simulink model "semi_active_suspension_mr_damper_full_vehicle"  (R2022b)
settings: Solver=ode1be  StartTime=0.0  StopTime=120  FixedStep=0.001  RelTol=1e-3
model workspace (MAT data in the model file):
  D_common1 = 500
  I_common = 50
  P_common = 4000
  a1 = 1.6
  a2 = 1.6
  a3 = 1.4
  a4 = 1.4
  filter_coefficient = 2000
  mr_damper_base_damping = 500
  s1 = 0.78
  s2 = 0.78
  s3 = 0.79
  s4 = 0.79
libraries: slpidlib x4
settings Model: Creator=giris  LastModifiedBy=giris

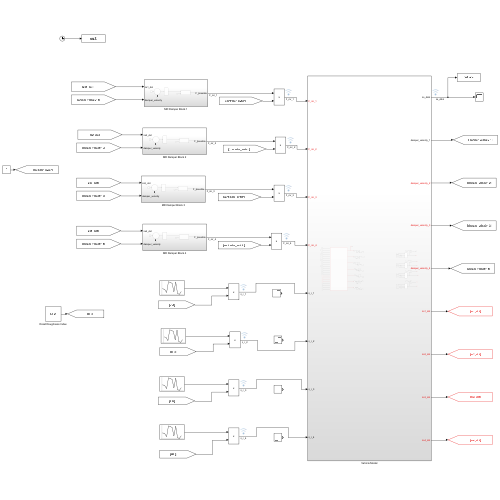
[thumbnail: Simulink's stored preview of the top-level diagram]
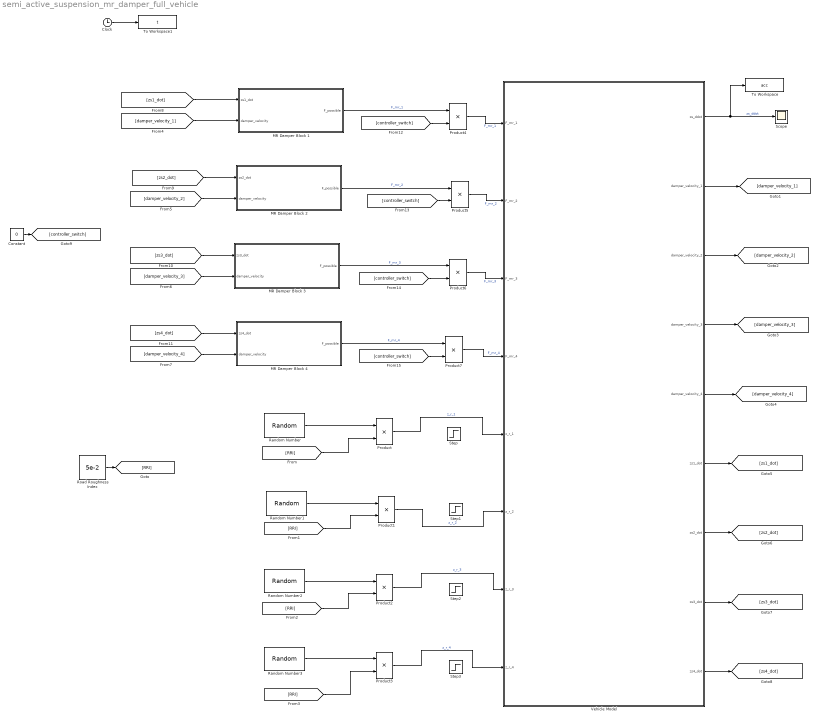
== system semi_active_suspension_mr_damper_full_vehicle ==
  Clock : Clock
  Constant : Constant  Value=0
  MR Damper Block 1 : Subsystem
  MR Damper Block 2 : Subsystem
  MR Damper Block 3 : Subsystem
  MR Damper Block 4 : Subsystem
  Product{,1..7} (8 alike) : Product
  Random Number : RandomNumber  SampleTime=0.01
  Random Number1 : RandomNumber  Seed=1  SampleTime=0.01
  Random Number2 : RandomNumber  Seed=2  SampleTime=0.01
  Random Number3 : RandomNumber  Seed=3  SampleTime=0.01
  Road Roughness Index : Constant  Value=5e-2
  Scope : Scope
  Step : Step  After=0.01  SampleTime=0
  Step1 : Step  After=0.01  SampleTime=0
  Step2 : Step  Time=1.135  After=0.01  SampleTime=0
  Step3 : Step  Time=1.135  After=0.01  SampleTime=0
  To Workspace : ToWorkspace  VariableName=acc  SaveFormat=Timeseries  SampleTime=-1
  To Workspace1 : ToWorkspace  VariableName=t  SaveFormat=Timeseries  SampleTime=-1
  Vehicle Model : Subsystem
  wires:
  MR Damper Block 3/1(F_possible) -> Product6/1  "F_mr_3"
  Random Number2/1 -> Product2/1
  Random Number/1 -> Product/1
  MR Damper Block 4/1(F_possible) -> Product7/1  "F_mr_4"
  Random Number1/1 -> Product1/1
  Random Number3/1 -> Product3/1
  MR Damper Block 1/1(F_possible) -> Product4/1  "F_mr_1"
  MR Damper Block 2/1(F_possible) -> Product5/1  "F_mr_2"
  Vehicle Model/1(zs_ddot) -> To Workspace/1, Scope/1  "zs_ddot"
  Road Roughness Index/1 -> [RRI]
  [RRI] -> Product/2
  [RRI] -> Product2/2
  [RRI] -> Product3/2
  [RRI] -> Product1/2
  Vehicle Model/5(damper_velocity_4) -> [damper_velocity_4]
  Vehicle Model/4(damper_velocity_3) -> [damper_velocity_3]
  Vehicle Model/3(damper_velocity_2) -> [damper_velocity_2]
  [damper_velocity_1] -> MR Damper Block 1/2(damper_velocity)
  [damper_velocity_2] -> MR Damper Block 2/2(damper_velocity)
  [damper_velocity_3] -> MR Damper Block 3/2(damper_velocity)
  [damper_velocity_4] -> MR Damper Block 4/2(damper_velocity)
  Vehicle Model/6(zs1_dot) -> [zs1_dot]
  Vehicle Model/7(zs2_dot) -> [zs2_dot]
  Vehicle Model/8(zs3_dot) -> [zs3_dot]
  Vehicle Model/9(zs4_dot) -> [zs4_dot]
  [zs1_dot] -> MR Damper Block 1/1(zs1_dot)
  [zs2_dot] -> MR Damper Block 2/1(zs2_dot)
  [zs3_dot] -> MR Damper Block 3/1(zs3_dot)
  [zs4_dot] -> MR Damper Block 4/1(zs4_dot)
  Product4/1 -> Vehicle Model/1(F_mr_1)  "F_mr_1"
  Product5/1 -> Vehicle Model/2(F_mr_2)  "F_mr_2"
  Product6/1 -> Vehicle Model/3(F_mr_3)  "F_mr_3"
  Product7/1 -> Vehicle Model/4(F_mr_4)  "F_mr_4"
  Constant/1 -> [controller_switch]
  [controller_switch] -> Product4/2
  [controller_switch] -> Product5/2
  [controller_switch] -> Product6/2
  [controller_switch] -> Product7/2
  Vehicle Model/2(damper_velocity_1) -> [damper_velocity_1]
  Clock/1 -> To Workspace1/1
  Product/1 -> Vehicle Model/5(z_r_1)  "z_r_1"
  Product1/1 -> Vehicle Model/6(z_r_2)  "z_r_2"
  Product2/1 -> Vehicle Model/7(z_r_3)  "z_r_3"
  Product3/1 -> Vehicle Model/8(z_r_4)  "z_r_4"

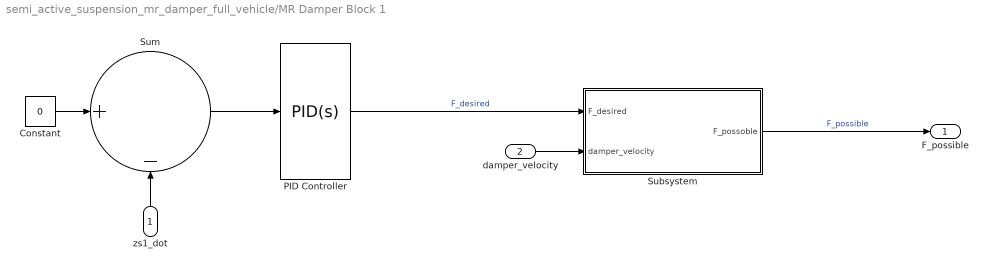
== system semi_active_suspension_mr_damper_full_vehicle/MR Damper Block 1 ==
  zs1_dot : Inport
  damper_velocity : Inport  Port=2
  Constant : Constant  Value=0
  PID Controller : slpidlib/PID Controller  Controller=PID  Form=Parallel  TimeDomain=Continuous-time  UseExternalTs=off  SampleTime=-1  IntegratorMethod=Forward Euler  FilterMethod=Forward Euler  ControllerParametersSource=internal  P=P_common  I=I_common  UseKiTs=off  D=D_common1  N=filter_coefficient  UseFilter=on  TunerSelectOption=Transfer Function Based (PID Tuner App)  InitialConditionSource=internal  InitialConditionForIntegrator=0  InitialConditionForFilter=0  DifferentiatorICPrevScaledInput=0  ExternalReset=none  TrackingMode=off  Kt=1  LimitOutput=off  SatLimitsSource=internal  UpperSaturationLimit=inf  LowerSaturationLimit=-inf  LinearizeAsGain=on  AntiWindupMode=none  Kb=1  LimitIntegrator=off  UpperIntegratorSaturationLimit=inf  LowerIntegratorSaturationLimit=-inf  POutMin=[]  POutMax=[]  IOutMin=[]  IOutMax=[]  DOutMin=[]  DOutMax=[]  NOutMin=[]  NOutMax=[]  SumOutMin=[]  SumOutMax=[]  SaturationOutMin=[]  SaturationOutMax=[]  PParamMin=[]  PParamMax=[]  IParamMin=[]  IParamMax=[]  DParamMin=[]  DParamMax=[]  NParamMin=[]  NParamMax=[]  KbParamMin=[]  KbParamMax=[]  KtParamMin=[]  KtParamMax=[]  KbOutMin=[]  KbOutMax=[]  KtOutMin=[]  KtOutMax=[]  IntegratorOutMin=[]  IntegratorOutMax=[]  FilterOutMin=[]  FilterOutMax=[]  SumI1OutMin=[]  SumI1OutMax=[]  SumI2OutMin=[]  SumI2OutMax=[]  SumI3OutMin=[]  SumI3OutMax=[]  SumI4OutMin=[]  SumI4OutMax=[]  SumDOutMin=[]  SumDOutMax=[]  DifferentiatorOutMin=[]  DifferentiatorOutMax=[]  FilterDiffOutCoefMin=[]  FilterDiffOutCoefMax=[]  ReciprocalOutMin=[]  ReciprocalOutMax=[]  SumDenOutMin=[]  SumDenOutMax=[]  SumNumOutMin=[]  SumNumOutMax=[]  DivideOutMin=[]  DivideOutMax=[]  UdiffTsProdOutMin=[]  UdiffTsProdOutMax=[]  NTsProdOutMin=[]  NTsProdOutMax=[]  UintegralTsProdOutMin=[]  UintegralTsProdOutMax=[]  UngainTsProdOutMin=[]  UngainTsProdOutMax=[]  ClampingZeroOutDataTypeStr=Inherit: Inherit via back propagation  ClampingZeroOutMin=[]  ClampingZeroOutMax=[]  FilterDenConstantOutDataTypeStr=Inherit: Inherit via back propagation  FilterDenConstantOutMin=[]  FilterDenConstantOutMax=[]  PCopyOutDataTypeStr=Inherit: Inherit via back propagation  PCopyOutMin=[]  PCopyOutMax=[]  NCopyOutDataTypeStr=Inherit: Inherit via back propagation  NCopyOutMin=[]  NCopyOutMax=[]  IntegratorContinuousStateAttributes=''  IntegratorStateMustResolveToSignalObject=off  IntegratorRTWStateStorageClass=Auto  FilterContinuousStateAttributes=''  FilterStateMustResolveToSignalObject=off  FilterRTWStateStorageClass=Auto  ParallelPVariant=InternalParameters  IdealPVariant=Disabled  IVariant=InternalParameters  DVariant=InternalParameters  IntegratorVariant=Continuous  SatVariant=Disabled  AWVariant=Passthrough  PCopyVariant=Disabled  TRVariant=Disabled  FdbkBlocksVariant=Forward  IdealPFdbkVariant=Disabled  SatFdbkVariant=Disabled  DerivativeFilterVariant=ContFilter  NVariant=InternalParameters  NCopyVariant=Disabled  FilterICVariant=InternalICsFilter  IntegratorICVariant=InternalICs  ExternalResetVariant=Disabled  TRSumVariant=Passthrough  SumFdbkVariant=Disabled  SumVariant=Sum_PID  TsampFilterVariant=InternalTs  TsampNgainVariant=Passthrough  TsampIntegralVariant=Passthrough  ExternalSaturationOutDataTypeStr=Inherit: Same as second input
  Subsystem : Subsystem
  Sum : Sum  Inputs=|+-
  F_possible : Outport
  wires:
  PID Controller/1 -> Subsystem/1(F_desired)  "F_desired"
  Subsystem/1(F_possoble) -> F_possible/1  "F_possible"
  Sum/1 -> PID Controller/1
  Constant/1 -> Sum/1
  zs1_dot/1 -> Sum/2
  damper_velocity/1 -> Subsystem/2(damper_velocity)

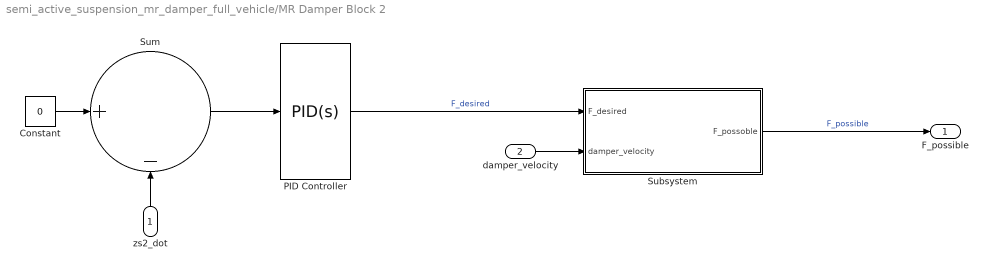
== system semi_active_suspension_mr_damper_full_vehicle/MR Damper Block 2 ==
  zs2_dot : Inport
  damper_velocity : Inport  Port=2
  Constant : Constant  Value=0
  PID Controller : slpidlib/PID Controller  Controller=PID  Form=Parallel  TimeDomain=Continuous-time  UseExternalTs=off  SampleTime=-1  IntegratorMethod=Forward Euler  FilterMethod=Forward Euler  ControllerParametersSource=internal  P=P_common  I=I_common  UseKiTs=off  D=D_common1  N=filter_coefficient  UseFilter=on  TunerSelectOption=Transfer Function Based (PID Tuner App)  InitialConditionSource=internal  InitialConditionForIntegrator=0  InitialConditionForFilter=0  DifferentiatorICPrevScaledInput=0  ExternalReset=none  TrackingMode=off  Kt=1  LimitOutput=off  SatLimitsSource=internal  UpperSaturationLimit=inf  LowerSaturationLimit=-inf  LinearizeAsGain=on  AntiWindupMode=none  Kb=1  LimitIntegrator=off  UpperIntegratorSaturationLimit=inf  LowerIntegratorSaturationLimit=-inf  POutMin=[]  POutMax=[]  IOutMin=[]  IOutMax=[]  DOutMin=[]  DOutMax=[]  NOutMin=[]  NOutMax=[]  SumOutMin=[]  SumOutMax=[]  SaturationOutMin=[]  SaturationOutMax=[]  PParamMin=[]  PParamMax=[]  IParamMin=[]  IParamMax=[]  DParamMin=[]  DParamMax=[]  NParamMin=[]  NParamMax=[]  KbParamMin=[]  KbParamMax=[]  KtParamMin=[]  KtParamMax=[]  KbOutMin=[]  KbOutMax=[]  KtOutMin=[]  KtOutMax=[]  IntegratorOutMin=[]  IntegratorOutMax=[]  FilterOutMin=[]  FilterOutMax=[]  SumI1OutMin=[]  SumI1OutMax=[]  SumI2OutMin=[]  SumI2OutMax=[]  SumI3OutMin=[]  SumI3OutMax=[]  SumI4OutMin=[]  SumI4OutMax=[]  SumDOutMin=[]  SumDOutMax=[]  DifferentiatorOutMin=[]  DifferentiatorOutMax=[]  FilterDiffOutCoefMin=[]  FilterDiffOutCoefMax=[]  ReciprocalOutMin=[]  ReciprocalOutMax=[]  SumDenOutMin=[]  SumDenOutMax=[]  SumNumOutMin=[]  SumNumOutMax=[]  DivideOutMin=[]  DivideOutMax=[]  UdiffTsProdOutMin=[]  UdiffTsProdOutMax=[]  NTsProdOutMin=[]  NTsProdOutMax=[]  UintegralTsProdOutMin=[]  UintegralTsProdOutMax=[]  UngainTsProdOutMin=[]  UngainTsProdOutMax=[]  ClampingZeroOutDataTypeStr=Inherit: Inherit via back propagation  ClampingZeroOutMin=[]  ClampingZeroOutMax=[]  FilterDenConstantOutDataTypeStr=Inherit: Inherit via back propagation  FilterDenConstantOutMin=[]  FilterDenConstantOutMax=[]  PCopyOutDataTypeStr=Inherit: Inherit via back propagation  PCopyOutMin=[]  PCopyOutMax=[]  NCopyOutDataTypeStr=Inherit: Inherit via back propagation  NCopyOutMin=[]  NCopyOutMax=[]  IntegratorContinuousStateAttributes=''  IntegratorStateMustResolveToSignalObject=off  IntegratorRTWStateStorageClass=Auto  FilterContinuousStateAttributes=''  FilterStateMustResolveToSignalObject=off  FilterRTWStateStorageClass=Auto  ParallelPVariant=InternalParameters  IdealPVariant=Disabled  IVariant=InternalParameters  DVariant=InternalParameters  IntegratorVariant=Continuous  SatVariant=Disabled  AWVariant=Passthrough  PCopyVariant=Disabled  TRVariant=Disabled  FdbkBlocksVariant=Forward  IdealPFdbkVariant=Disabled  SatFdbkVariant=Disabled  DerivativeFilterVariant=ContFilter  NVariant=InternalParameters  NCopyVariant=Disabled  FilterICVariant=InternalICsFilter  IntegratorICVariant=InternalICs  ExternalResetVariant=Disabled  TRSumVariant=Passthrough  SumFdbkVariant=Disabled  SumVariant=Sum_PID  TsampFilterVariant=InternalTs  TsampNgainVariant=Passthrough  TsampIntegralVariant=Passthrough  ExternalSaturationOutDataTypeStr=Inherit: Same as second input
  Subsystem : Subsystem
  Sum : Sum  Inputs=|+-
  F_possible : Outport
  wires:
  damper_velocity/1 -> Subsystem/2(damper_velocity)
  zs2_dot/1 -> Sum/2
  Constant/1 -> Sum/1
  Sum/1 -> PID Controller/1
  Subsystem/1(F_possoble) -> F_possible/1  "F_possible"
  PID Controller/1 -> Subsystem/1(F_desired)  "F_desired"

== system semi_active_suspension_mr_damper_full_vehicle/MR Damper Block 3 ==
  zs3_dot : Inport
  damper_velocity : Inport  Port=2
  Constant : Constant  Value=0
  PID Controller : slpidlib/PID Controller  Controller=PID  Form=Parallel  TimeDomain=Continuous-time  UseExternalTs=off  SampleTime=-1  IntegratorMethod=Forward Euler  FilterMethod=Forward Euler  ControllerParametersSource=internal  P=P_common  I=I_common  UseKiTs=off  D=D_common1  N=filter_coefficient  UseFilter=on  TunerSelectOption=Transfer Function Based (PID Tuner App)  InitialConditionSource=internal  InitialConditionForIntegrator=0  InitialConditionForFilter=0  DifferentiatorICPrevScaledInput=0  ExternalReset=none  TrackingMode=off  Kt=1  LimitOutput=off  SatLimitsSource=internal  UpperSaturationLimit=inf  LowerSaturationLimit=-inf  LinearizeAsGain=on  AntiWindupMode=none  Kb=1  LimitIntegrator=off  UpperIntegratorSaturationLimit=inf  LowerIntegratorSaturationLimit=-inf  POutMin=[]  POutMax=[]  IOutMin=[]  IOutMax=[]  DOutMin=[]  DOutMax=[]  NOutMin=[]  NOutMax=[]  SumOutMin=[]  SumOutMax=[]  SaturationOutMin=[]  SaturationOutMax=[]  PParamMin=[]  PParamMax=[]  IParamMin=[]  IParamMax=[]  DParamMin=[]  DParamMax=[]  NParamMin=[]  NParamMax=[]  KbParamMin=[]  KbParamMax=[]  KtParamMin=[]  KtParamMax=[]  KbOutMin=[]  KbOutMax=[]  KtOutMin=[]  KtOutMax=[]  IntegratorOutMin=[]  IntegratorOutMax=[]  FilterOutMin=[]  FilterOutMax=[]  SumI1OutMin=[]  SumI1OutMax=[]  SumI2OutMin=[]  SumI2OutMax=[]  SumI3OutMin=[]  SumI3OutMax=[]  SumI4OutMin=[]  SumI4OutMax=[]  SumDOutMin=[]  SumDOutMax=[]  DifferentiatorOutMin=[]  DifferentiatorOutMax=[]  FilterDiffOutCoefMin=[]  FilterDiffOutCoefMax=[]  ReciprocalOutMin=[]  ReciprocalOutMax=[]  SumDenOutMin=[]  SumDenOutMax=[]  SumNumOutMin=[]  SumNumOutMax=[]  DivideOutMin=[]  DivideOutMax=[]  UdiffTsProdOutMin=[]  UdiffTsProdOutMax=[]  NTsProdOutMin=[]  NTsProdOutMax=[]  UintegralTsProdOutMin=[]  UintegralTsProdOutMax=[]  UngainTsProdOutMin=[]  UngainTsProdOutMax=[]  ClampingZeroOutDataTypeStr=Inherit: Inherit via back propagation  ClampingZeroOutMin=[]  ClampingZeroOutMax=[]  FilterDenConstantOutDataTypeStr=Inherit: Inherit via back propagation  FilterDenConstantOutMin=[]  FilterDenConstantOutMax=[]  PCopyOutDataTypeStr=Inherit: Inherit via back propagation  PCopyOutMin=[]  PCopyOutMax=[]  NCopyOutDataTypeStr=Inherit: Inherit via back propagation  NCopyOutMin=[]  NCopyOutMax=[]  IntegratorContinuousStateAttributes=''  IntegratorStateMustResolveToSignalObject=off  IntegratorRTWStateStorageClass=Auto  FilterContinuousStateAttributes=''  FilterStateMustResolveToSignalObject=off  FilterRTWStateStorageClass=Auto  ParallelPVariant=InternalParameters  IdealPVariant=Disabled  IVariant=InternalParameters  DVariant=InternalParameters  IntegratorVariant=Continuous  SatVariant=Disabled  AWVariant=Passthrough  PCopyVariant=Disabled  TRVariant=Disabled  FdbkBlocksVariant=Forward  IdealPFdbkVariant=Disabled  SatFdbkVariant=Disabled  DerivativeFilterVariant=ContFilter  NVariant=InternalParameters  NCopyVariant=Disabled  FilterICVariant=InternalICsFilter  IntegratorICVariant=InternalICs  ExternalResetVariant=Disabled  TRSumVariant=Passthrough  SumFdbkVariant=Disabled  SumVariant=Sum_PID  TsampFilterVariant=InternalTs  TsampNgainVariant=Passthrough  TsampIntegralVariant=Passthrough  ExternalSaturationOutDataTypeStr=Inherit: Same as second input
  Subsystem : Subsystem
  Sum : Sum  Inputs=|+-
  F_possible : Outport
  wires:
  PID Controller/1 -> Subsystem/1(F_desired)  "F_desired"
  Subsystem/1(F_possoble) -> F_possible/1  "F_possible"
  Sum/1 -> PID Controller/1
  Constant/1 -> Sum/1
  zs3_dot/1 -> Sum/2
  damper_velocity/1 -> Subsystem/2(damper_velocity)

== system semi_active_suspension_mr_damper_full_vehicle/MR Damper Block 4 ==
  zs4_dot : Inport
  damper_velocity : Inport  Port=2
  Constant : Constant  Value=0
  PID Controller : slpidlib/PID Controller  Controller=PID  Form=Parallel  TimeDomain=Continuous-time  UseExternalTs=off  SampleTime=-1  IntegratorMethod=Forward Euler  FilterMethod=Forward Euler  ControllerParametersSource=internal  P=P_common  I=I_common  UseKiTs=off  D=D_common1  N=filter_coefficient  UseFilter=on  TunerSelectOption=Transfer Function Based (PID Tuner App)  InitialConditionSource=internal  InitialConditionForIntegrator=0  InitialConditionForFilter=0  DifferentiatorICPrevScaledInput=0  ExternalReset=none  TrackingMode=off  Kt=1  LimitOutput=off  SatLimitsSource=internal  UpperSaturationLimit=inf  LowerSaturationLimit=-inf  LinearizeAsGain=on  AntiWindupMode=none  Kb=1  LimitIntegrator=off  UpperIntegratorSaturationLimit=inf  LowerIntegratorSaturationLimit=-inf  POutMin=[]  POutMax=[]  IOutMin=[]  IOutMax=[]  DOutMin=[]  DOutMax=[]  NOutMin=[]  NOutMax=[]  SumOutMin=[]  SumOutMax=[]  SaturationOutMin=[]  SaturationOutMax=[]  PParamMin=[]  PParamMax=[]  IParamMin=[]  IParamMax=[]  DParamMin=[]  DParamMax=[]  NParamMin=[]  NParamMax=[]  KbParamMin=[]  KbParamMax=[]  KtParamMin=[]  KtParamMax=[]  KbOutMin=[]  KbOutMax=[]  KtOutMin=[]  KtOutMax=[]  IntegratorOutMin=[]  IntegratorOutMax=[]  FilterOutMin=[]  FilterOutMax=[]  SumI1OutMin=[]  SumI1OutMax=[]  SumI2OutMin=[]  SumI2OutMax=[]  SumI3OutMin=[]  SumI3OutMax=[]  SumI4OutMin=[]  SumI4OutMax=[]  SumDOutMin=[]  SumDOutMax=[]  DifferentiatorOutMin=[]  DifferentiatorOutMax=[]  FilterDiffOutCoefMin=[]  FilterDiffOutCoefMax=[]  ReciprocalOutMin=[]  ReciprocalOutMax=[]  SumDenOutMin=[]  SumDenOutMax=[]  SumNumOutMin=[]  SumNumOutMax=[]  DivideOutMin=[]  DivideOutMax=[]  UdiffTsProdOutMin=[]  UdiffTsProdOutMax=[]  NTsProdOutMin=[]  NTsProdOutMax=[]  UintegralTsProdOutMin=[]  UintegralTsProdOutMax=[]  UngainTsProdOutMin=[]  UngainTsProdOutMax=[]  ClampingZeroOutDataTypeStr=Inherit: Inherit via back propagation  ClampingZeroOutMin=[]  ClampingZeroOutMax=[]  FilterDenConstantOutDataTypeStr=Inherit: Inherit via back propagation  FilterDenConstantOutMin=[]  FilterDenConstantOutMax=[]  PCopyOutDataTypeStr=Inherit: Inherit via back propagation  PCopyOutMin=[]  PCopyOutMax=[]  NCopyOutDataTypeStr=Inherit: Inherit via back propagation  NCopyOutMin=[]  NCopyOutMax=[]  IntegratorContinuousStateAttributes=''  IntegratorStateMustResolveToSignalObject=off  IntegratorRTWStateStorageClass=Auto  FilterContinuousStateAttributes=''  FilterStateMustResolveToSignalObject=off  FilterRTWStateStorageClass=Auto  ParallelPVariant=InternalParameters  IdealPVariant=Disabled  IVariant=InternalParameters  DVariant=InternalParameters  IntegratorVariant=Continuous  SatVariant=Disabled  AWVariant=Passthrough  PCopyVariant=Disabled  TRVariant=Disabled  FdbkBlocksVariant=Forward  IdealPFdbkVariant=Disabled  SatFdbkVariant=Disabled  DerivativeFilterVariant=ContFilter  NVariant=InternalParameters  NCopyVariant=Disabled  FilterICVariant=InternalICsFilter  IntegratorICVariant=InternalICs  ExternalResetVariant=Disabled  TRSumVariant=Passthrough  SumFdbkVariant=Disabled  SumVariant=Sum_PID  TsampFilterVariant=InternalTs  TsampNgainVariant=Passthrough  TsampIntegralVariant=Passthrough  ExternalSaturationOutDataTypeStr=Inherit: Same as second input
  Subsystem : Subsystem
  Sum : Sum  Inputs=|+-
  F_possible : Outport
  wires:
  damper_velocity/1 -> Subsystem/2(damper_velocity)
  zs4_dot/1 -> Sum/2
  Constant/1 -> Sum/1
  Sum/1 -> PID Controller/1
  Subsystem/1(F_possoble) -> F_possible/1  "F_possible"
  PID Controller/1 -> Subsystem/1(F_desired)  "F_desired"

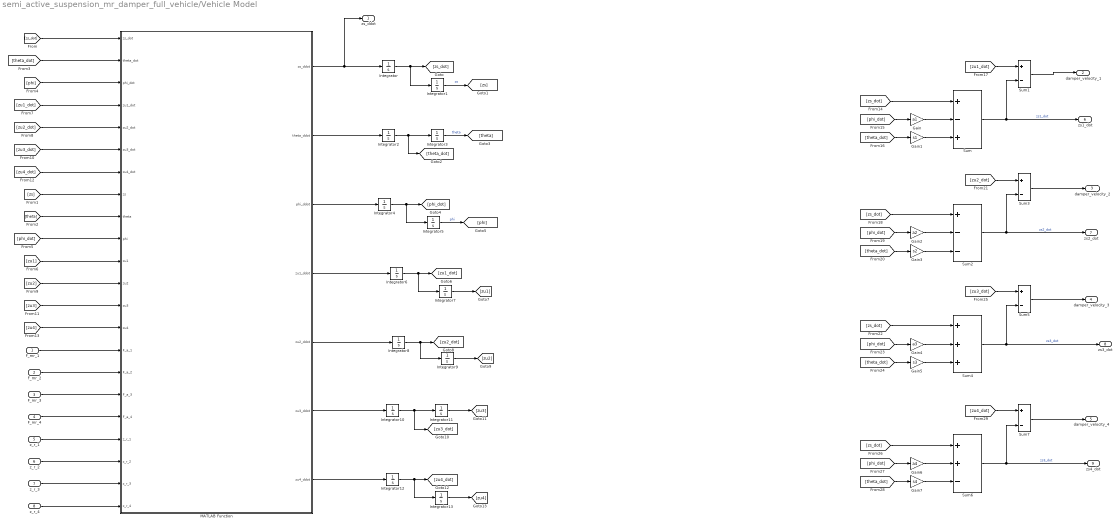
== system semi_active_suspension_mr_damper_full_vehicle/Vehicle Model ==
  F_mr_1 : Inport
  F_mr_2 : Inport  Port=2
  F_mr_3 : Inport  Port=3
  F_mr_4 : Inport  Port=4
  z_r_1 : Inport  Port=5
  z_r_2 : Inport  Port=6
  z_r_3 : Inport  Port=7
  z_r_4 : Inport  Port=8
  Gain : Gain  Gain=a1
  Gain1 : Gain  Gain=s1
  Gain2 : Gain  Gain=a2
  Gain3 : Gain  Gain=s2
  Gain4 : Gain  Gain=a3
  Gain5 : Gain  Gain=s3
  Gain6 : Gain  Gain=a4
  Gain7 : Gain  Gain=s4
  Integrator{,1..13} (14 alike) : Integrator
  MATLAB Function : MATLAB Function  TreatAsAtomicUnit=on
  Sum : Sum  Inputs=+-+
  Sum{1,3,5,7} (4 alike) : Sum  Inputs=+-
  Sum2 : Sum  Inputs=+--
  Sum4 : Sum  Inputs=+++
  Sum6 : Sum  Inputs=++-
  zs_ddot : Outport
  damper_velocity_1 : Outport  Port=2
  damper_velocity_2 : Outport  Port=3
  damper_velocity_3 : Outport  Port=4
  damper_velocity_4 : Outport  Port=5
  zs1_dot : Outport  Port=6
  zs2_dot : Outport  Port=7
  zs3_dot : Outport  Port=8
  zs4_dot : Outport  Port=9
  wires:
  Integrator3/1 -> [theta]  "theta"
  [zu2_dot] -> MATLAB Function/5(zu2_dot)
  [zu3_dot] -> MATLAB Function/6(zu3_dot)
  [theta_dot] -> MATLAB Function/2(theta_dot)
  z_r_3/1 -> MATLAB Function/21(z_r_3)
  [zs_dot] -> MATLAB Function/1(zs_dot)
  [phi] -> MATLAB Function/3(phi_dot)
  z_r_2/1 -> MATLAB Function/20(z_r_2)
  [zs] -> MATLAB Function/8(zs)
  Integrator12/1 -> Integrator13/1, [zu4_dot]
  [zu1_dot] -> MATLAB Function/4(zu1_dot)
  Integrator8/1 -> [zu2_dot], Integrator9/1
  [zu4_dot] -> MATLAB Function/7(zu4_dot)
  [zu3] -> MATLAB Function/13(zu3)
  [theta] -> MATLAB Function/9(theta)
  [phi_dot] -> MATLAB Function/10(phi)
  Integrator11/1 -> [zu3]
  [zu1] -> MATLAB Function/11(zu1)
  [zu2] -> MATLAB Function/12(zu2)
  [zu4] -> MATLAB Function/14(zu4)
  z_r_1/1 -> MATLAB Function/19(z_r_1)
  z_r_4/1 -> MATLAB Function/22(z_r_4)
  MATLAB Function/1(zs_ddot) -> zs_ddot/1, Integrator/1
  MATLAB Function/2(theta_ddot) -> Integrator2/1
  MATLAB Function/3(phi_ddot) -> Integrator4/1
  MATLAB Function/4(zu1_ddot) -> Integrator6/1
  MATLAB Function/5(zu2_ddot) -> Integrator8/1
  MATLAB Function/6(zu3_ddot) -> Integrator10/1
  Integrator6/1 -> Integrator7/1, [zu1_dot]
  MATLAB Function/7(zu4_ddot) -> Integrator12/1
  Integrator/1 -> Integrator1/1, [zs_dot]
  Integrator2/1 -> [theta_dot], Integrator3/1
  Integrator4/1 -> [phi_dot], Integrator5/1
  Integrator7/1 -> [zu1]
  Integrator10/1 -> [zu3_dot], Integrator11/1
  Integrator1/1 -> [zs]  "zs"
  Integrator5/1 -> [phi]  "phi"
  Integrator9/1 -> [zu2]
  Integrator13/1 -> [zu4]
  F_mr_1/1 -> MATLAB Function/15(F_a_1)
  F_mr_2/1 -> MATLAB Function/16(F_a_2)
  F_mr_3/1 -> MATLAB Function/17(F_a_3)
  F_mr_4/1 -> MATLAB Function/18(F_a_4)
  [zs_dot] -> Sum/1
  [phi_dot] -> Gain/1
  Gain/1 -> Sum/2
  [theta_dot] -> Gain1/1
  Gain1/1 -> Sum/3
  Sum/1 -> Sum1/2, zs1_dot/1  "zs1_dot"
  [zu1_dot] -> Sum1/1
  Sum1/1 -> damper_velocity_1/1
  Sum3/1 -> damper_velocity_2/1
  [zu2_dot] -> Sum3/1
  Sum2/1 -> zs2_dot/1, Sum3/2  "zs2_dot"
  Gain3/1 -> Sum2/3
  [theta_dot] -> Gain3/1
  Gain2/1 -> Sum2/2
  [phi_dot] -> Gain2/1
  [zs_dot] -> Sum2/1
  [zs_dot] -> Sum4/1
  [phi_dot] -> Gain4/1
  Gain4/1 -> Sum4/2
  [theta_dot] -> Gain5/1
  Gain5/1 -> Sum4/3
  Sum4/1 -> zs3_dot/1, Sum5/2  "zs3_dot"
  [zu3_dot] -> Sum5/1
  Sum5/1 -> damper_velocity_3/1
  Sum7/1 -> damper_velocity_4/1
  [zu4_dot] -> Sum7/1
  Sum6/1 -> zs4_dot/1, Sum7/2  "zs3_dot"
  Gain7/1 -> Sum6/3
  [theta_dot] -> Gain7/1
  Gain6/1 -> Sum6/2
  [phi_dot] -> Gain6/1
  [zs_dot] -> Sum6/1

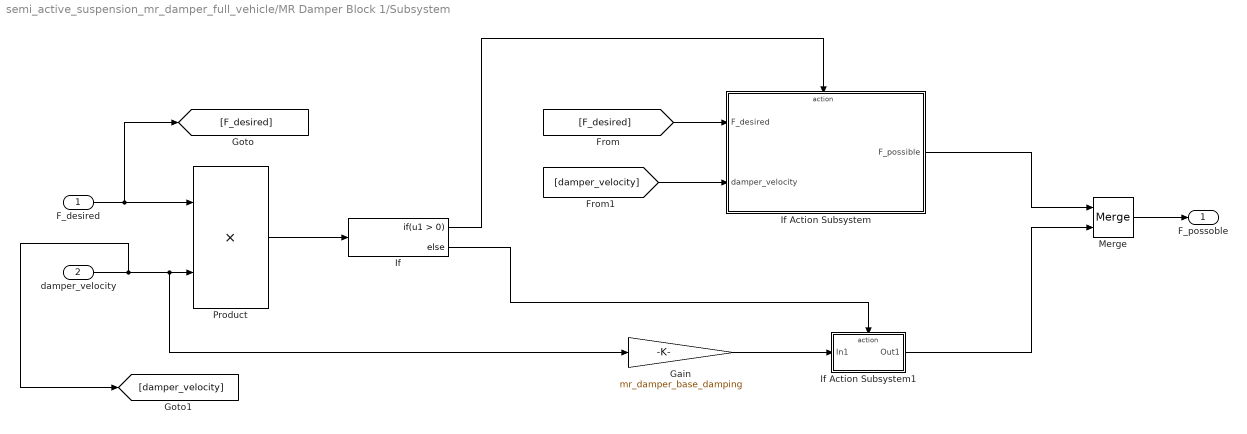
== system semi_active_suspension_mr_damper_full_vehicle/MR Damper Block 1/Subsystem ==
  F_desired : Inport
  damper_velocity : Inport  Port=2
  Gain : Gain  Gain=mr_damper_base_damping
  If : If
  If Action Subsystem : Subsystem  TreatAsAtomicUnit=on
  If Action Subsystem1 : Subsystem  TreatAsAtomicUnit=on
  Merge : Merge
  Product : Product
  F_possoble : Outport
  wires:
  F_desired/1 -> [F_desired], Product/1
  damper_velocity/1 -> [damper_velocity], Gain/1, Product/2
  Product/1 -> If/1
  If/1 -> If Action Subsystem/Action
  If Action Subsystem/1(F_possible) -> Merge/1
  Merge/1 -> F_possoble/1
  If/2 -> If Action Subsystem1/Action
  Gain/1 -> If Action Subsystem1/1(In1)
  If Action Subsystem1/1(Out1) -> Merge/2
  [F_desired] -> If Action Subsystem/1(F_desired)
  [damper_velocity] -> If Action Subsystem/2(damper_velocity)

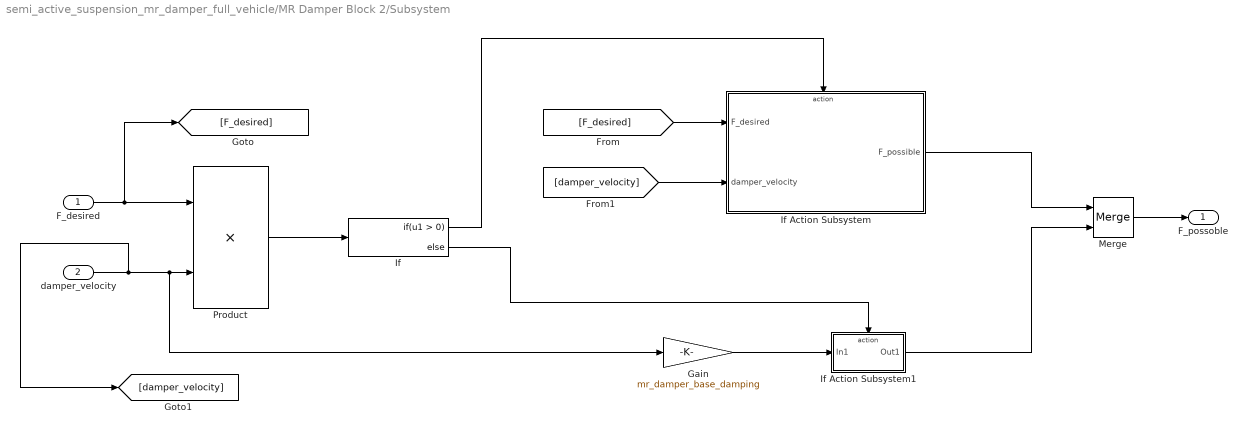
== system semi_active_suspension_mr_damper_full_vehicle/MR Damper Block 2/Subsystem ==
  F_desired : Inport
  damper_velocity : Inport  Port=2
  Gain : Gain  Gain=mr_damper_base_damping
  If : If
  If Action Subsystem : Subsystem  TreatAsAtomicUnit=on
  If Action Subsystem1 : Subsystem  TreatAsAtomicUnit=on
  Merge : Merge
  Product : Product
  F_possoble : Outport
  wires:
  [damper_velocity] -> If Action Subsystem/2(damper_velocity)
  [F_desired] -> If Action Subsystem/1(F_desired)
  If Action Subsystem1/1(Out1) -> Merge/2
  Gain/1 -> If Action Subsystem1/1(In1)
  If/2 -> If Action Subsystem1/Action
  Merge/1 -> F_possoble/1
  If Action Subsystem/1(F_possible) -> Merge/1
  If/1 -> If Action Subsystem/Action
  Product/1 -> If/1
  damper_velocity/1 -> Product/2, Gain/1, [damper_velocity]
  F_desired/1 -> Product/1, [F_desired]

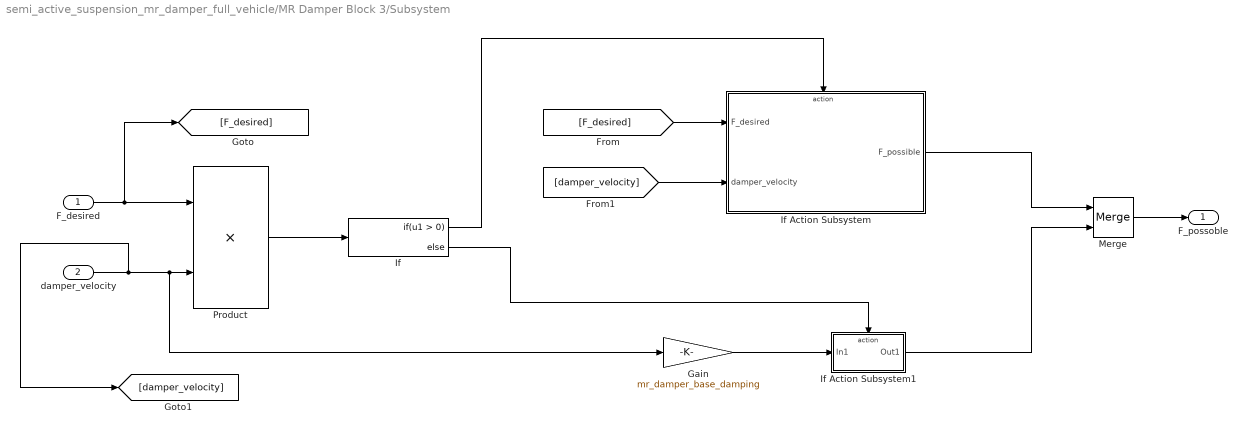
== system semi_active_suspension_mr_damper_full_vehicle/MR Damper Block 3/Subsystem ==
  F_desired : Inport
  damper_velocity : Inport  Port=2
  Gain : Gain  Gain=mr_damper_base_damping
  If : If
  If Action Subsystem : Subsystem  TreatAsAtomicUnit=on
  If Action Subsystem1 : Subsystem  TreatAsAtomicUnit=on
  Merge : Merge
  Product : Product
  F_possoble : Outport
  wires:
  F_desired/1 -> [F_desired], Product/1
  damper_velocity/1 -> [damper_velocity], Gain/1, Product/2
  Product/1 -> If/1
  If/1 -> If Action Subsystem/Action
  If Action Subsystem/1(F_possible) -> Merge/1
  Merge/1 -> F_possoble/1
  If/2 -> If Action Subsystem1/Action
  Gain/1 -> If Action Subsystem1/1(In1)
  If Action Subsystem1/1(Out1) -> Merge/2
  [F_desired] -> If Action Subsystem/1(F_desired)
  [damper_velocity] -> If Action Subsystem/2(damper_velocity)

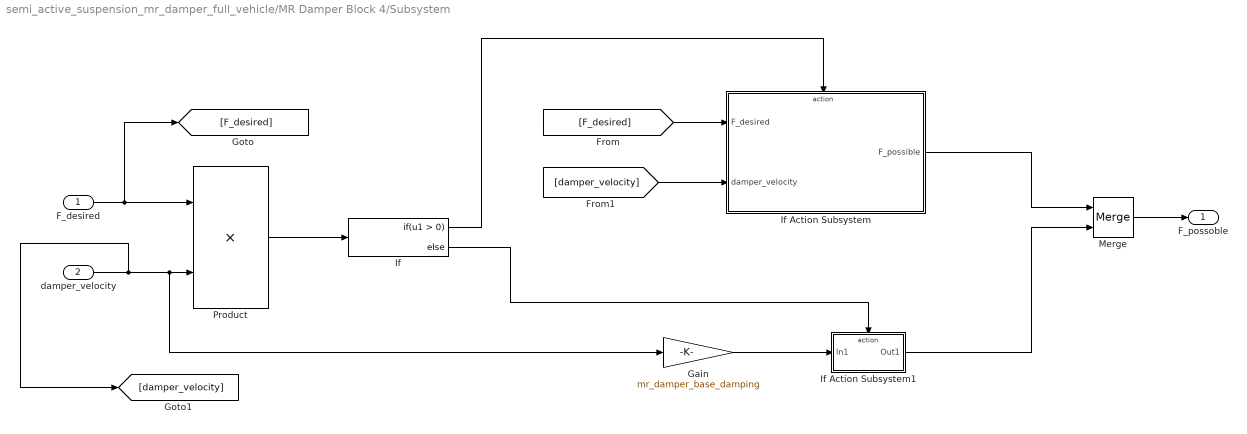
== system semi_active_suspension_mr_damper_full_vehicle/MR Damper Block 4/Subsystem ==
  F_desired : Inport
  damper_velocity : Inport  Port=2
  Gain : Gain  Gain=mr_damper_base_damping
  If : If
  If Action Subsystem : Subsystem  TreatAsAtomicUnit=on
  If Action Subsystem1 : Subsystem  TreatAsAtomicUnit=on
  Merge : Merge
  Product : Product
  F_possoble : Outport
  wires:
  [damper_velocity] -> If Action Subsystem/2(damper_velocity)
  [F_desired] -> If Action Subsystem/1(F_desired)
  If Action Subsystem1/1(Out1) -> Merge/2
  Gain/1 -> If Action Subsystem1/1(In1)
  If/2 -> If Action Subsystem1/Action
  Merge/1 -> F_possoble/1
  If Action Subsystem/1(F_possible) -> Merge/1
  If/1 -> If Action Subsystem/Action
  Product/1 -> If/1
  damper_velocity/1 -> Product/2, Gain/1, [damper_velocity]
  F_desired/1 -> Product/1, [F_desired]

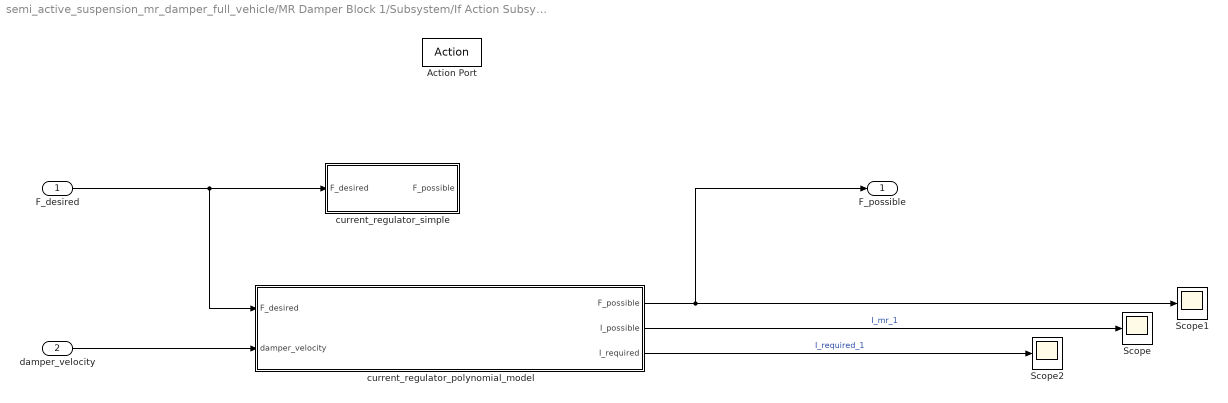
== system semi_active_suspension_mr_damper_full_vehicle/MR Damper Block 1/Subsystem/If Action Subsystem ==
  F_desired : Inport
  damper_velocity : Inport  Port=2
  Action Port : ActionPort  ActionPortLabel=if(u1 > 0)
  Scope : Scope
  Scope1 : Scope
  Scope2 : Scope
  current_regulator_polynomial_model : MATLAB Function  TreatAsAtomicUnit=on
  current_regulator_simple : MATLAB Function  TreatAsAtomicUnit=on
  F_possible : Outport
  wires:
  damper_velocity/1 -> current_regulator_polynomial_model/2(damper_velocity)
  F_desired/1 -> current_regulator_polynomial_model/1(F_desired), current_regulator_simple/1(F_desired)
  current_regulator_polynomial_model/1(F_possible) -> F_possible/1, Scope1/1
  current_regulator_polynomial_model/2(I_possible) -> Scope/1  "I_mr_1"
  current_regulator_polynomial_model/3(I_required) -> Scope2/1  "I_required_1"

== system semi_active_suspension_mr_damper_full_vehicle/MR Damper Block 1/Subsystem/If Action Subsystem1 ==
  In1 : Inport
  Action Port : ActionPort  ActionPortLabel=else
  Out1 : Outport
  wires:
  In1/1 -> Out1/1

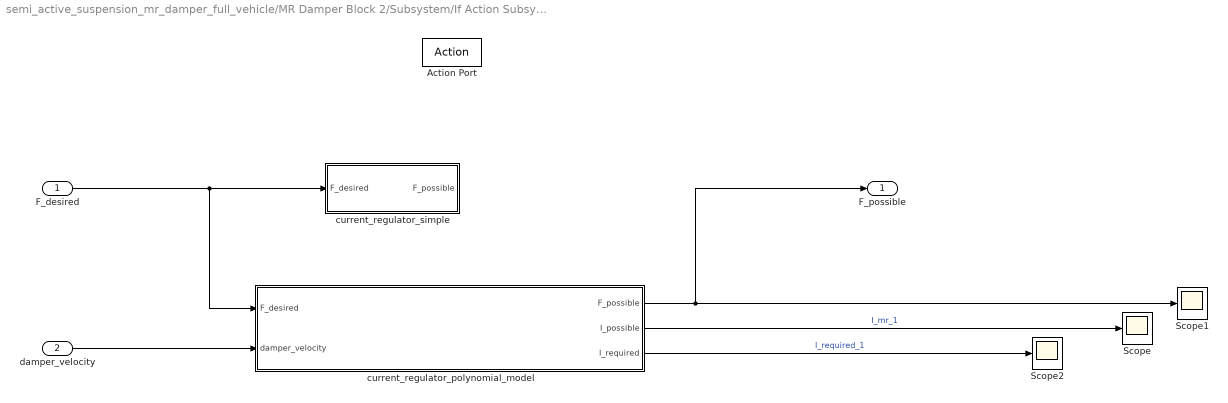
== system semi_active_suspension_mr_damper_full_vehicle/MR Damper Block 2/Subsystem/If Action Subsystem ==
  F_desired : Inport
  damper_velocity : Inport  Port=2
  Action Port : ActionPort  ActionPortLabel=if(u1 > 0)
  Scope : Scope
  Scope1 : Scope
  Scope2 : Scope
  current_regulator_polynomial_model : MATLAB Function  TreatAsAtomicUnit=on
  current_regulator_simple : MATLAB Function  TreatAsAtomicUnit=on
  F_possible : Outport
  wires:
  current_regulator_polynomial_model/3(I_required) -> Scope2/1  "I_required_1"
  current_regulator_polynomial_model/2(I_possible) -> Scope/1  "I_mr_1"
  current_regulator_polynomial_model/1(F_possible) -> Scope1/1, F_possible/1
  F_desired/1 -> current_regulator_simple/1(F_desired), current_regulator_polynomial_model/1(F_desired)
  damper_velocity/1 -> current_regulator_polynomial_model/2(damper_velocity)

== system semi_active_suspension_mr_damper_full_vehicle/MR Damper Block 2/Subsystem/If Action Subsystem1 ==
  In1 : Inport
  Action Port : ActionPort  ActionPortLabel=else
  Out1 : Outport
  wires:
  In1/1 -> Out1/1

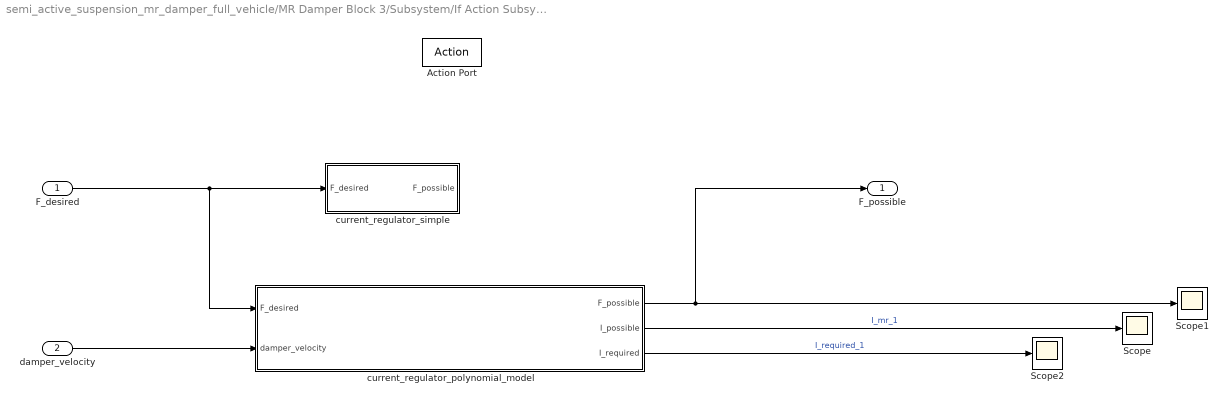
== system semi_active_suspension_mr_damper_full_vehicle/MR Damper Block 3/Subsystem/If Action Subsystem ==
  F_desired : Inport
  damper_velocity : Inport  Port=2
  Action Port : ActionPort  ActionPortLabel=if(u1 > 0)
  Scope : Scope
  Scope1 : Scope
  Scope2 : Scope
  current_regulator_polynomial_model : MATLAB Function  TreatAsAtomicUnit=on
  current_regulator_simple : MATLAB Function  TreatAsAtomicUnit=on
  F_possible : Outport
  wires:
  damper_velocity/1 -> current_regulator_polynomial_model/2(damper_velocity)
  F_desired/1 -> current_regulator_polynomial_model/1(F_desired), current_regulator_simple/1(F_desired)
  current_regulator_polynomial_model/1(F_possible) -> F_possible/1, Scope1/1
  current_regulator_polynomial_model/2(I_possible) -> Scope/1  "I_mr_1"
  current_regulator_polynomial_model/3(I_required) -> Scope2/1  "I_required_1"

== system semi_active_suspension_mr_damper_full_vehicle/MR Damper Block 3/Subsystem/If Action Subsystem1 ==
  In1 : Inport
  Action Port : ActionPort  ActionPortLabel=else
  Out1 : Outport
  wires:
  In1/1 -> Out1/1

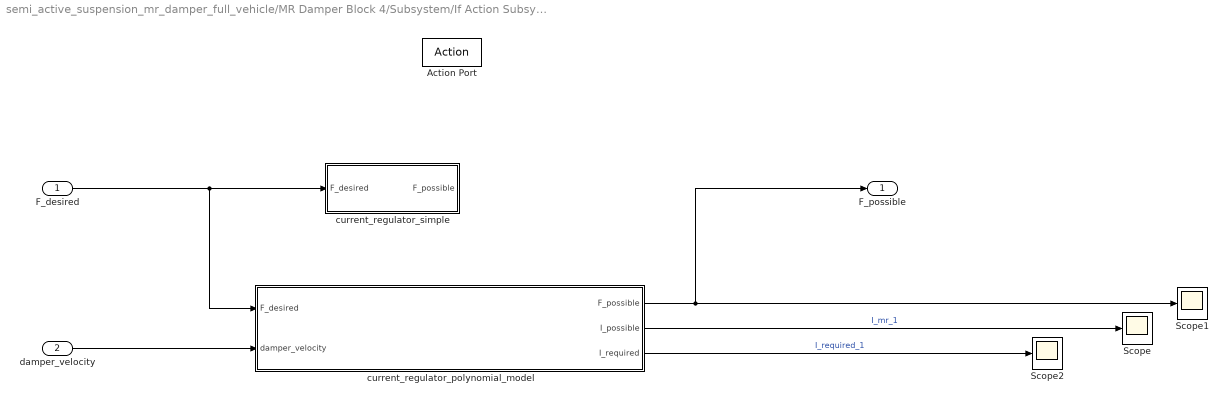
== system semi_active_suspension_mr_damper_full_vehicle/MR Damper Block 4/Subsystem/If Action Subsystem ==
  F_desired : Inport
  damper_velocity : Inport  Port=2
  Action Port : ActionPort  ActionPortLabel=if(u1 > 0)
  Scope : Scope
  Scope1 : Scope
  Scope2 : Scope
  current_regulator_polynomial_model : MATLAB Function  TreatAsAtomicUnit=on
  current_regulator_simple : MATLAB Function  TreatAsAtomicUnit=on
  F_possible : Outport
  wires:
  current_regulator_polynomial_model/3(I_required) -> Scope2/1  "I_required_1"
  current_regulator_polynomial_model/2(I_possible) -> Scope/1  "I_mr_1"
  current_regulator_polynomial_model/1(F_possible) -> Scope1/1, F_possible/1
  F_desired/1 -> current_regulator_simple/1(F_desired), current_regulator_polynomial_model/1(F_desired)
  damper_velocity/1 -> current_regulator_polynomial_model/2(damper_velocity)

== system semi_active_suspension_mr_damper_full_vehicle/MR Damper Block 4/Subsystem/If Action Subsystem1 ==
  In1 : Inport
  Action Port : ActionPort  ActionPortLabel=else
  Out1 : Outport
  wires:
  In1/1 -> Out1/1

== matlab function semi_active_suspension_mr_damper_full_vehicle/MR Damper Block 4/Subsystem/If Action Subsystem/current_regulator_polynomial_model ==
  data: F_desired input; F_possible output; damper_velocity input; I_possible output; I_required output
function [F_possible, I_possible, I_required] = current_regulator_polynomial_model(F_desired, damper_velocity)


v = damper_velocity*1;
I_max = 15;

c0 = -659.4;
c1 = 8.995;
c2 = 0.1062;
c3 = -1.584e-4;
c4 = -5.908e-6;
c5 = 1.137e-9;
c6 = 1.087e-10;
c7 = 0;
c8 = 0;
c9 = 0;
c10 = 0;
c11 = 0;


I_required = (F_desired)/(1000*(0*c0*v^0 + c1*v^1 + c2*v^2 + c3*v^3 + c4*v^4 + c5*v^5 + c6*v^6 + c7*v^7 + c8*v^8 + c9*v^9 + c10*v^10 + c11*v^11));

if abs(I_required) > I_max
    I_possible = I_max;
else
    I_possible = I_required;
end


F_possible = (1000*(0*c0*v^0 + c1*v^1 + c2*v^2 + c3*v^3 + c4*v^4 + c5*v^5 + c6*v^6 + c7*v^7 + c8*v^8 + c9*v^9 + c10*v^10 + c11*v^11))*I_possible;

== matlab function semi_active_suspension_mr_damper_full_vehicle/MR Damper Block 4/Subsystem/If Action Subsystem/current_regulator_simple ==
  data: F_desired input; F_possible output
function F_possible = current_regulator_simple(F_desired)

cs = 1000; % N/A

I_required = F_desired/cs;

I_max = 3;

if abs(I_required) > I_max

    I_possible = sign(F_desired)*I_max;

else

    I_possible = I_required;

end

F_possible = I_possible * cs;

== matlab function semi_active_suspension_mr_damper_full_vehicle/Vehicle Model/MATLAB Function ==
  data: zs_dot input; theta_dot input; phi_dot input; zu1_dot input; zu2_dot input; zu3_dot input; zu4_dot input; zs input; theta input; phi input; zu1 input; zu2 input; zu3 input; zu4 input; F_a_1 input; F_a_2 input; F_a_3 input; F_a_4 input; z_r_1 input; zs_ddot output; z_r_2 input; z_r_3 input; z_r_4 input; theta_ddot output; phi_ddot output; zu1_ddot output; zu2_ddot output; zu3_ddot output; zu4_ddot output
function [zs_ddot, theta_ddot, phi_ddot, zu1_ddot, zu2_ddot, zu3_ddot, zu4_ddot] = ...
            ...
            fcn(zs_dot, theta_dot, phi_dot, zu1_dot, zu2_dot, zu3_dot, zu4_dot, zs, theta, phi, zu1, zu2, zu3, zu4, ...
                                                                                       F_a_1, F_a_2, F_a_3, F_a_4, ...
                                                                                       z_r_1, z_r_2, z_r_3, z_r_4)


% State - variable initialization
% zs_dot = X(1);
% theta_dot = X(2);
% phi_dot = X(3);
% zu1_dot = X(4);
% zu2_dot = X(5);
% zu3_dot = X(6);
% zu4_dot = X(7);
% 
% zs = X(8);
% theta = X(9);
% phi = X(10);
% zu1 = X(11);
% zu2 = X(12);
% zu3 = X(13);
% zu4 = X(14);

%% Vehicle & Component Inputs
% Quarter Car Component Inputs
d_s = 7250;       % Ns/m
m_s = 4*510;       % kg
Ixx = 200;
Iyy = 1700;
m_a = 60;        % kg
k_s = 1*52500;     % N/m
k_t = 200000;    % N/m
d_t = 1*100;
k_arb = 103000; % Nm/rad


a1 = 1.6;
a2 = 1.6;
a3 = 1.4;
a4 = 1.4;

s1 = 0.78;
s2 = 0.78;
s3 = 0.79;
s4 = 0.79;

arb_switch = 0;


%% Chassis Corner Displacements
zs1 = zs - a1*phi + s1*theta;
zs2 = zs - a2*phi - s2*theta;
zs3 = zs + a3*phi + s3*theta;
zs4 = zs + a4*phi - s4*theta;



zs1_dot = zs_dot - a1*phi_dot + s1*theta_dot;
zs2_dot = zs_dot - a2*phi_dot - s2*theta_dot;
zs3_dot = zs_dot + a3*phi_dot + s3*theta_dot;
zs4_dot = zs_dot + a4*phi_dot - s4*theta_dot;


%% Suspension Displacement & Velocity

% NOTE: Needed for ARB twist calculation
Delta_s1 = zu1 - zs1;
Delta_s2 = zu2 - zs2;
Delta_s3 = zu3 - zs3;
Delta_s4 = zu4 - zs4;

Delta_dot_s1 = zu1_dot - zs1_dot;
Delta_dot_s2 = zu2_dot - zs1_dot;
Delta_dot_s3 = zu3_dot - zs3_dot;
Delta_dot_s4 = zu4_dot - zs4_dot;

% ARB twist
torsion_arb_f = atan((Delta_s1 - Delta_s2)/(s1 + s2));
torsion_arb_r = atan((Delta_s3 - Delta_s4)/(s3 + s4));


%% Force Calculations


% ARB Force Calculation
F_arb_f = arb_switch * k_arb * torsion_arb_f;
F_arb_r = arb_switch * k_arb * torsion_arb_r;

F_s_1 = k_s*(Delta_s1) + d_s*(Delta_dot_s1) + F_a_1 + F_arb_f/2;
F_s_2 = k_s*(Delta_s2) + d_s*(Delta_dot_s2) + F_a_2 - F_arb_f/2;
F_s_3 = k_s*(Delta_s3) + d_s*(Delta_dot_s3) + F_a_3 + F_arb_r/2;
F_s_4 = k_s*(Delta_s4) + d_s*(Delta_dot_s4) + F_a_4 - F_arb_r/2;

F_t_1 = k_t*(z_r_1 - zu1) + d_t*( - zu1_dot);
F_t_2 = k_t*(z_r_2 - zu2) + d_t*( - zu2_dot);
F_t_3 = k_t*(z_r_3 - zu3) + d_t*( - zu3_dot);
F_t_4 = k_t*(z_r_4 - zu4) + d_t*( - zu4_dot);


%% System Matrices

M = [m_s 0   0   0   0   0   0;
     0   Ixx 0   0   0   0   0;
     0   0   Iyy 0   0   0   0;
     0   0   0   m_a 0   0   0;
     0   0   0   0   m_a 0   0;
     0   0   0   0   0   m_a 0;
     0   0   0   0   0   0   m_a];


f_qd_q_u = [F_s_1 + F_s_2 + F_s_3 + F_s_4;
            s1*F_s_1 - s2*F_s_2 + s3*F_s_3 - s4*F_s_4;
           -a1*F_s_1 - a2*F_s_2 + a3*F_s_3 + a4*F_s_4;
           -F_s_1 + F_t_1;
           -F_s_2 + F_t_2;
           -F_s_3 + F_t_3;
           -F_s_4 + F_t_4];




Q_ddot = M\f_qd_q_u;

zs_ddot = Q_ddot(1);
theta_ddot = Q_ddot(2);
phi_ddot = Q_ddot(3);
zu1_ddot = Q_ddot(4);
zu2_ddot = Q_ddot(5);
zu3_ddot = Q_ddot(6);
zu4_ddot = Q_ddot(7);

== matlab function semi_active_suspension_mr_damper_full_vehicle/MR Damper Block 1/Subsystem/If Action Subsystem/current_regulator_polynomial_model ==
  data: F_desired input; F_possible output; damper_velocity input; I_possible output; I_required output
function [F_possible, I_possible, I_required] = current_regulator_polynomial_model(F_desired, damper_velocity)


v = damper_velocity*1;
I_max = 15;

c0 = -659.4;
c1 = 8.995;
c2 = 0.1062;
c3 = -1.584e-4;
c4 = -5.908e-6;
c5 = 1.137e-9;
c6 = 1.087e-10;
c7 = 0;
c8 = 0;
c9 = 0;
c10 = 0;
c11 = 0;


I_required = (F_desired)/(1000*(0*c0*v^0 + c1*v^1 + c2*v^2 + c3*v^3 + c4*v^4 + c5*v^5 + c6*v^6 + c7*v^7 + c8*v^8 + c9*v^9 + c10*v^10 + c11*v^11));

if abs(I_required) > I_max
    I_possible = I_max;
else
    I_possible = I_required;
end


F_possible = (1000*(0*c0*v^0 + c1*v^1 + c2*v^2 + c3*v^3 + c4*v^4 + c5*v^5 + c6*v^6 + c7*v^7 + c8*v^8 + c9*v^9 + c10*v^10 + c11*v^11))*I_possible;

== matlab function semi_active_suspension_mr_damper_full_vehicle/MR Damper Block 1/Subsystem/If Action Subsystem/current_regulator_simple ==
  data: F_desired input; F_possible output
function F_possible = current_regulator_simple(F_desired)

cs = 1000; % N/A

I_required = F_desired/cs;

I_max = 3;

if abs(I_required) > I_max

    I_possible = sign(F_desired)*I_max;

else

    I_possible = I_required;

end

F_possible = I_possible * cs;

== matlab function semi_active_suspension_mr_damper_full_vehicle/MR Damper Block 2/Subsystem/If Action Subsystem/current_regulator_polynomial_model ==
  data: F_desired input; F_possible output; damper_velocity input; I_possible output; I_required output
function [F_possible, I_possible, I_required] = current_regulator_polynomial_model(F_desired, damper_velocity)


v = damper_velocity*1;
I_max = 15;

c0 = -659.4;
c1 = 8.995;
c2 = 0.1062;
c3 = -1.584e-4;
c4 = -5.908e-6;
c5 = 1.137e-9;
c6 = 1.087e-10;
c7 = 0;
c8 = 0;
c9 = 0;
c10 = 0;
c11 = 0;


I_required = (F_desired)/(1000*(0*c0*v^0 + c1*v^1 + c2*v^2 + c3*v^3 + c4*v^4 + c5*v^5 + c6*v^6 + c7*v^7 + c8*v^8 + c9*v^9 + c10*v^10 + c11*v^11));

if abs(I_required) > I_max
    I_possible = I_max;
else
    I_possible = I_required;
end


F_possible = (1000*(0*c0*v^0 + c1*v^1 + c2*v^2 + c3*v^3 + c4*v^4 + c5*v^5 + c6*v^6 + c7*v^7 + c8*v^8 + c9*v^9 + c10*v^10 + c11*v^11))*I_possible;

== matlab function semi_active_suspension_mr_damper_full_vehicle/MR Damper Block 2/Subsystem/If Action Subsystem/current_regulator_simple ==
  data: F_desired input; F_possible output
function F_possible = current_regulator_simple(F_desired)

cs = 1000; % N/A

I_required = F_desired/cs;

I_max = 3;

if abs(I_required) > I_max

    I_possible = sign(F_desired)*I_max;

else

    I_possible = I_required;

end

F_possible = I_possible * cs;

== matlab function semi_active_suspension_mr_damper_full_vehicle/MR Damper Block 3/Subsystem/If Action Subsystem/current_regulator_polynomial_model ==
  data: F_desired input; F_possible output; damper_velocity input; I_possible output; I_required output
function [F_possible, I_possible, I_required] = current_regulator_polynomial_model(F_desired, damper_velocity)


v = damper_velocity*1;
I_max = 15;

c0 = -659.4;
c1 = 8.995;
c2 = 0.1062;
c3 = -1.584e-4;
c4 = -5.908e-6;
c5 = 1.137e-9;
c6 = 1.087e-10;
c7 = 0;
c8 = 0;
c9 = 0;
c10 = 0;
c11 = 0;


I_required = (F_desired)/(1000*(0*c0*v^0 + c1*v^1 + c2*v^2 + c3*v^3 + c4*v^4 + c5*v^5 + c6*v^6 + c7*v^7 + c8*v^8 + c9*v^9 + c10*v^10 + c11*v^11));

if abs(I_required) > I_max
    I_possible = I_max;
else
    I_possible = I_required;
end


F_possible = (1000*(0*c0*v^0 + c1*v^1 + c2*v^2 + c3*v^3 + c4*v^4 + c5*v^5 + c6*v^6 + c7*v^7 + c8*v^8 + c9*v^9 + c10*v^10 + c11*v^11))*I_possible;

== matlab function semi_active_suspension_mr_damper_full_vehicle/MR Damper Block 3/Subsystem/If Action Subsystem/current_regulator_simple ==
  data: F_desired input; F_possible output
function F_possible = current_regulator_simple(F_desired)

cs = 1000; % N/A

I_required = F_desired/cs;

I_max = 3;

if abs(I_required) > I_max

    I_possible = sign(F_desired)*I_max;

else

    I_possible = I_required;

end

F_possible = I_possible * cs;
